simulink model "BlockDiagram1_0"  (R2025b)
settings: Solver=VariableStepAuto  StartTime=0.0  StopTime=10.0  RelTol=1e-3
settings Model: Creator=gruby  LastModifiedBy=gruby

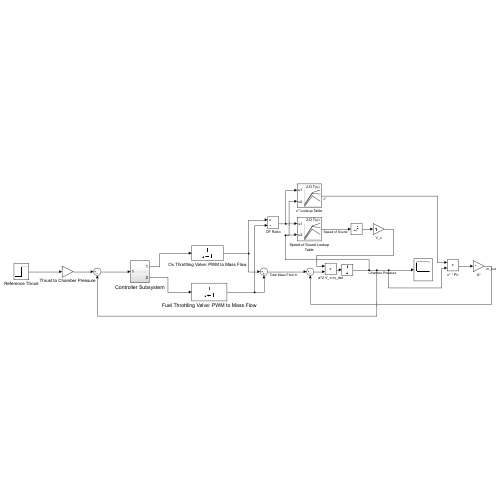
[thumbnail: Simulink's stored preview of the top-level diagram]
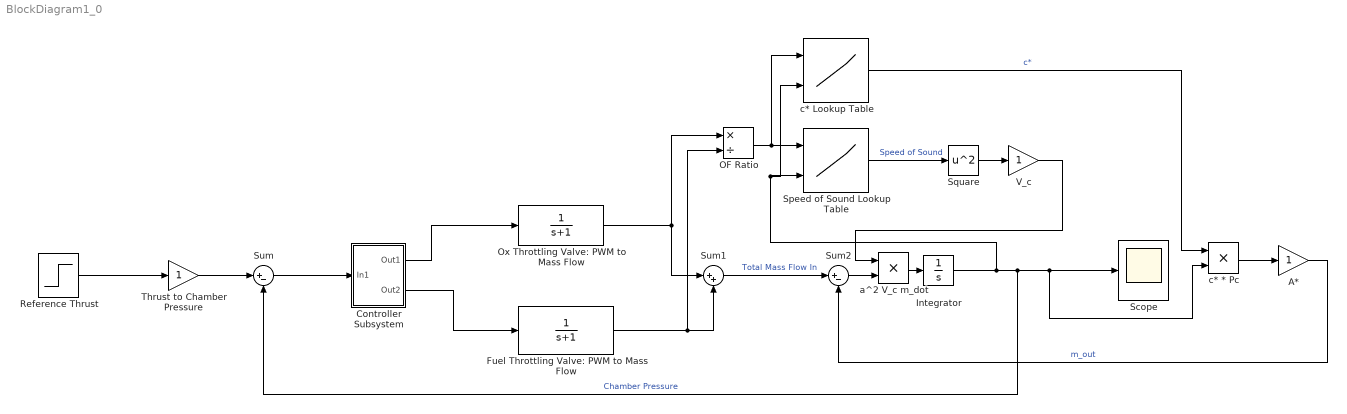
== system BlockDiagram1_0 ==
  A* : Gain
  Controller Subsystem : Subsystem
  Fuel Throttling Valve: PWM to Mass Flow : TransferFcn  Denominator=[1 1]
  Integrator : Integrator
  OF Ratio : Product  Inputs=*/
  Ox Throttling Valve: PWM to Mass Flow : TransferFcn  Denominator=[1 1]
  Reference Thrust : Step  SampleTime=0
  Scope : Scope
      settings: ActiveDisplayYMinimum=-1  ActiveDisplayYMaximum=1
  Speed of Sound Lookup Table : Lookup_n-D  BreakpointsForDimension1=[1:3]  BreakpointsForDimension2=[1:3]  InternalRulePriority=Speed  RndMeth=Simplest
      settings: InputPortMap=u0,u1
  Square : Math  Operator=square
  Sum : Sum  Inputs=|+-
  Sum1 : Sum  Inputs=|++
  Sum2 : Sum  Inputs=|+-
  Thrust to Chamber Pressure : Gain
  V_c : Gain
  a^2 V_c m_dot : Product
  c* * Pc : Product
  c* Lookup Table : Lookup_n-D  BreakpointsForDimension1=[1:3]  BreakpointsForDimension2=[1:3]  InternalRulePriority=Speed  RndMeth=Simplest
      settings: InputPortMap=u0,u1
  wires:
  Controller Subsystem/2(Out2) -> Fuel Throttling Valve: PWM to Mass Flow/1
  Integrator/1 -> Sum/2, c* * Pc/2, Scope/1, c* Lookup Table/2, Speed of Sound Lookup Table/2  "Chamber Pressure"
  Sum/1 -> Controller Subsystem/1(In1)
  Thrust to Chamber Pressure/1 -> Sum/1
  Reference Thrust/1 -> Thrust to Chamber Pressure/1
  Controller Subsystem/1(Out1) -> Ox Throttling Valve: PWM to Mass Flow/1
  Fuel Throttling Valve: PWM to Mass Flow/1 -> Sum1/2, OF Ratio/2
  Ox Throttling Valve: PWM to Mass Flow/1 -> OF Ratio/1, Sum1/1
  Sum1/1 -> Sum2/1  "Total Mass Flow In"
  OF Ratio/1 -> c* Lookup Table/1, Speed of Sound Lookup Table/1
  Speed of Sound Lookup Table/1 -> Square/1  "Speed of Sound"
  Square/1 -> V_c/1
  c* Lookup Table/1 -> c* * Pc/1  "c*"
  c* * Pc/1 -> A*/1
  A*/1 -> Sum2/2  "m_out"
  Sum2/1 -> a^2 V_c m_dot/2
  V_c/1 -> a^2 V_c m_dot/1
  a^2 V_c m_dot/1 -> Integrator/1

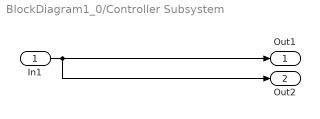
== system BlockDiagram1_0/Controller Subsystem ==
  In1 : Inport
  Out1 : Outport
  Out2 : Outport  Port=2
  wires:
  In1/1 -> Out2/1, Out1/1
